simulink model "untitled1"  (R2019b)
settings: Solver=VariableStepAuto  StartTime=0.0  StopTime=1  RelTol=1e-3
libraries: simulink x2, AveragingFilter x1
settings Model: Creator=Nick  LastModifiedBy=Nick

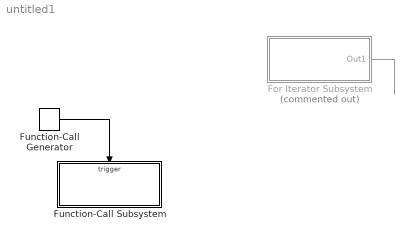
== system untitled1 ==
  For Iterator Subsystem : Subsystem  Commented=on  TreatAsAtomicUnit=on
  Function-Call Generator : simulink/Ports & Subsystems/Function-Call Generator  sample_time=0.00002  numberOfIterations=1
  Function-Call Subsystem : Subsystem  TreatAsAtomicUnit=on
  wires:
  For Iterator Subsystem/1(Out1) -> ?
  Function-Call Generator/1 -> Function-Call Subsystem/Trigger

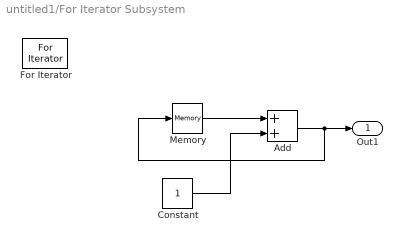
== system untitled1/For Iterator Subsystem ==
  Add : Sum
  Constant : Constant
  For Iterator : ForIterator  ResetStates=reset
  Memory : Memory  InheritSampleTime=on
  Out1 : Outport
  wires:
  Add/1 -> Memory/1, Out1/1
  Constant/1 -> Add/2
  Memory/1 -> Add/1

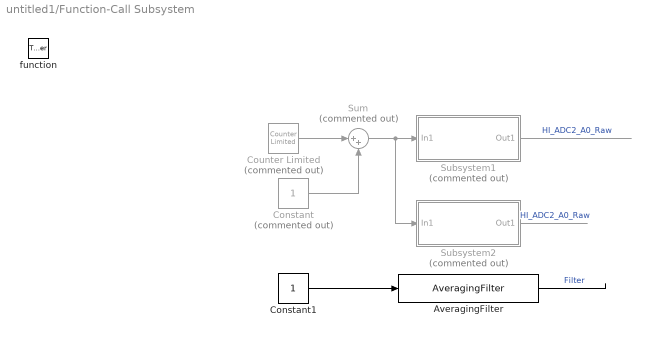
== system untitled1/Function-Call Subsystem ==
  function : TriggerPort  TriggerType=function-call  VariantControl=Variant
  AveragingFilter : AveragingFilter/AveragingFilter  factor=10
  Constant : Constant  Commented=on
  Constant1 : Constant
  Counter Limited : simulink/Sources/Counter Limited  Commented=on  uplimit=19  tsamp=-1
  Subsystem1 : Subsystem  Commented=on
  Subsystem2 : Subsystem  Commented=on
  Sum : Sum  Commented=on  Inputs=|++
  wires:
  Counter Limited/1 -> Sum/1
  Subsystem1/1(Out1) -> ?  "HI_ADC2_A0_Raw"
  Sum/1 -> Subsystem2/1(In1), Subsystem1/1(In1)
  Constant/1 -> Sum/2
  Subsystem2/1(Out1) -> ?  "HI_ADC2_A0_Raw"
  Constant1/1 -> AveragingFilter/1
  AveragingFilter/1 -> ?  "Filter"

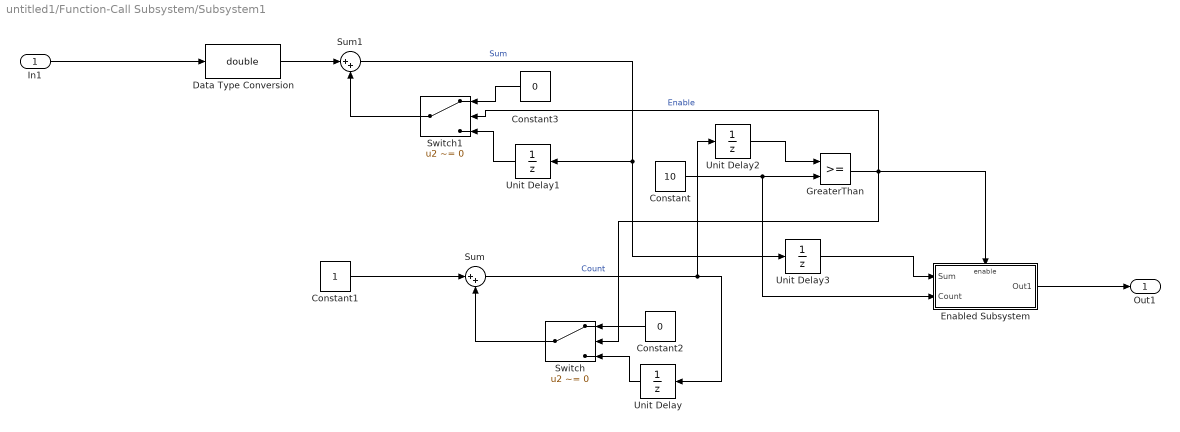
== system untitled1/Function-Call Subsystem/Subsystem1 ==
  In1 : Inport
  Constant : Constant  Value=10
  Constant1 : Constant
  Constant2 : Constant  Value=0
  Constant3 : Constant  Value=0
  Data Type Conversion : DataTypeConversion  OutDataTypeStr=double
  Enabled Subsystem : Subsystem  TreatAsAtomicUnit=on
  GreaterThan : RelationalOperator  OutDataTypeStr=boolean  RndMeth=Simplest
  Sum : Sum  Inputs=|++
  Sum1 : Sum  Inputs=|++
  Switch : Switch  Criteria=u2 ~= 0  Threshold=50
  Switch1 : Switch  Criteria=u2 ~= 0  Threshold=50
  Unit Delay{,1..3} (4 alike) : UnitDelay  SampleTime=-1  HasFrameUpgradeWarning=on
  Out1 : Outport
  wires:
  In1/1 -> Data Type Conversion/1
  Constant/1 -> Enabled Subsystem/2(Count), GreaterThan/2
  Sum1/1 -> Unit Delay3/1, Unit Delay1/1  "Sum"
  Sum/1 -> Unit Delay/1, Unit Delay2/1  "Count"
  GreaterThan/1 -> Switch1/2, Switch/2, Enabled Subsystem/Enable  "Enable"
  Constant1/1 -> Sum/1
  Unit Delay/1 -> Switch/3
  Constant2/1 -> Switch/1
  Switch/1 -> Sum/2
  Data Type Conversion/1 -> Sum1/1
  Unit Delay1/1 -> Switch1/3
  Constant3/1 -> Switch1/1
  Switch1/1 -> Sum1/2
  Unit Delay3/1 -> Enabled Subsystem/1(Sum)
  Unit Delay2/1 -> GreaterThan/1
  Enabled Subsystem/1(Out1) -> Out1/1

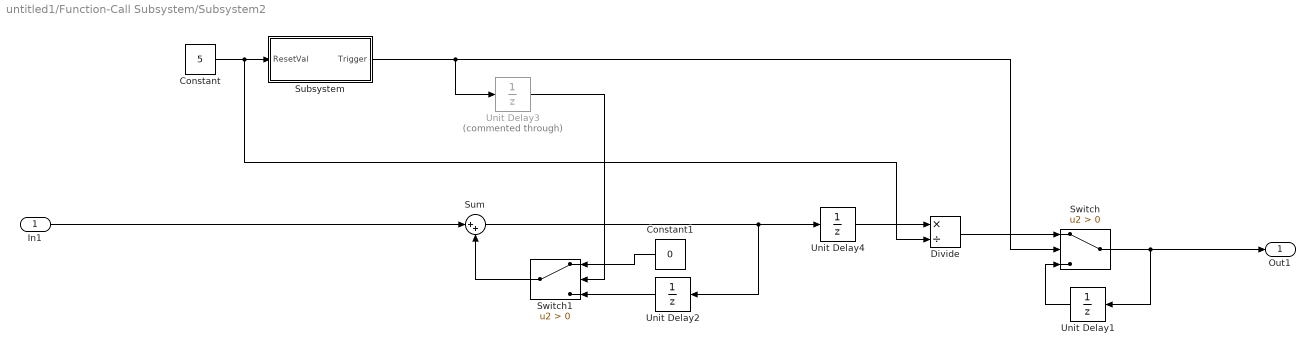
== system untitled1/Function-Call Subsystem/Subsystem2 ==
  In1 : Inport
  Constant : Constant  Value=5
  Constant1 : Constant  Value=0
  Divide : Product  Inputs=*/
  Subsystem : Subsystem
  Sum : Sum  Inputs=|++
  Switch : Switch  Criteria=u2 > Threshold
  Switch1 : Switch  Criteria=u2 > Threshold
  Unit Delay1 : UnitDelay  SampleTime=-1  HasFrameUpgradeWarning=on
  Unit Delay2 : UnitDelay  SampleTime=-1  HasFrameUpgradeWarning=on
  Unit Delay3 : UnitDelay  Commented=through  SampleTime=-1  HasFrameUpgradeWarning=on
  Unit Delay4 : UnitDelay  SampleTime=-1  HasFrameUpgradeWarning=on
  Out1 : Outport
  wires:
  Switch/1 -> Unit Delay1/1, Out1/1
  Unit Delay1/1 -> Switch/3
  Constant/1 -> Divide/2, Subsystem/1(ResetVal)
  Subsystem/1(Trigger) -> Unit Delay3/1, Switch/2
  In1/1 -> Sum/1
  Switch1/1 -> Sum/2
  Unit Delay2/1 -> Switch1/3
  Constant1/1 -> Switch1/1
  Divide/1 -> Switch/1
  Sum/1 -> Unit Delay4/1, Unit Delay2/1
  Unit Delay3/1 -> Switch1/2
  Unit Delay4/1 -> Divide/1

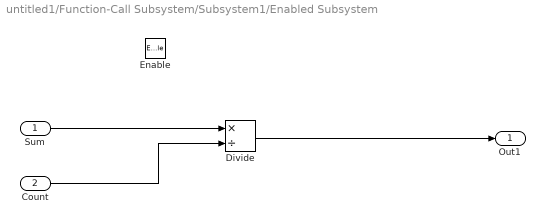
== system untitled1/Function-Call Subsystem/Subsystem1/Enabled Subsystem ==
  Sum : Inport
  Count : Inport  Port=2
  Enable : EnablePort
  Divide : Product  Inputs=*/
  Out1 : Outport
  wires:
  Sum/1 -> Divide/1
  Count/1 -> Divide/2
  Divide/1 -> Out1/1

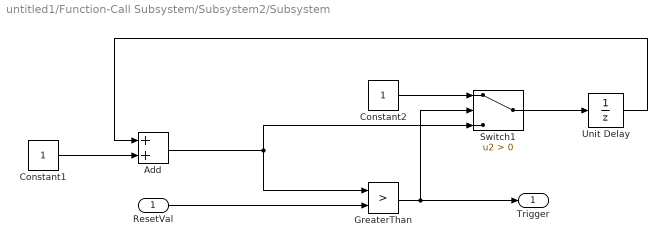
== system untitled1/Function-Call Subsystem/Subsystem2/Subsystem ==
  ResetVal : Inport
  Add : Sum
  Constant1 : Constant
  Constant2 : Constant
  GreaterThan : RelationalOperator  Operator=>  OutDataTypeStr=boolean  RndMeth=Simplest
  Switch1 : Switch  Criteria=u2 > Threshold
  Unit Delay : UnitDelay  SampleTime=-1  HasFrameUpgradeWarning=on
  Trigger : Outport
  wires:
  Add/1 -> GreaterThan/1, Switch1/3
  Unit Delay/1 -> Add/1
  GreaterThan/1 -> Trigger/1, Switch1/2
  Switch1/1 -> Unit Delay/1
  ResetVal/1 -> GreaterThan/2
  Constant2/1 -> Switch1/1
  Constant1/1 -> Add/2
